simulink subsystem "Torque_Actuated_Configuration_Space_Controller"  (R2021a)
settings: Solver=VariableStepAuto  StartTime=0.0  StopTime=10.0  RelTol=1e-3
undefined symbols (not defined in the file or in its folder): X, Y, Z
libraries: OpenManipulatorLib x5, sm_lib x4, nesl_utility x1
settings Model: Creator=USER  LastModifiedBy=USER

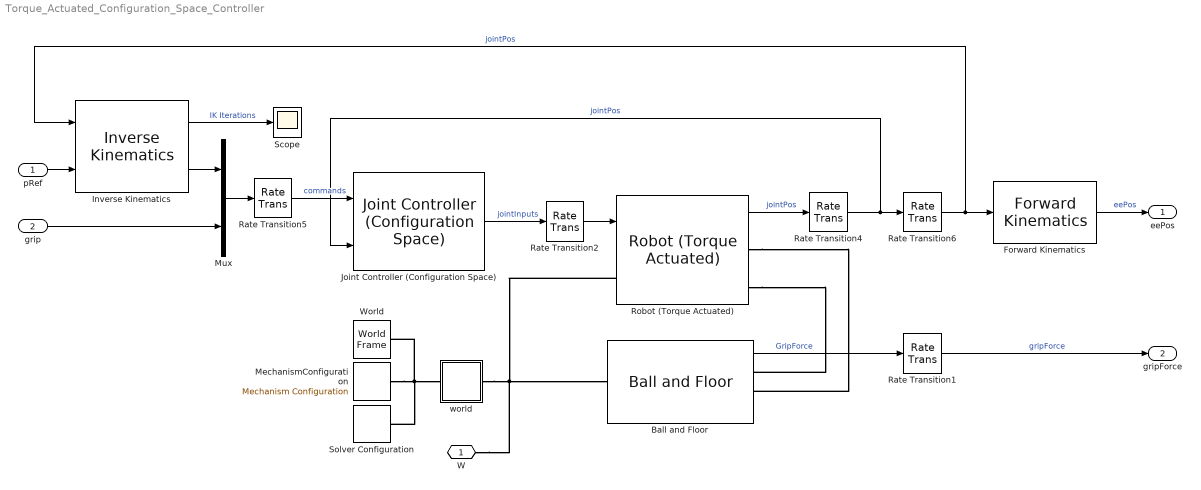
== system Torque_Actuated_Configuration_Space_Controller ==
  "pRef " : Inport
  grip : Inport  Port=2
  Ball and Floor : OpenManipulatorLib/Ball and Floor  PxPositionTargetValue=initPosX  PyPositionTargetValue=initPosY  PxVelocityTargetValue=initVelX  PyVelocityTargetValue=initVelY  PzPositionTargetValue=initPosZ  PzVelocityTargetValue=initVelZ
  Forward Kinematics : OpenManipulatorLib/Forward Kinematics  SystemSampleTime=-1  VariantActivationTime=update diagram  Latency=0  AutoFrameSizeCalculation=off
  Inverse Kinematics : OpenManipulatorLib/Inverse Kinematics  SystemSampleTime=-1  VariantActivationTime=update diagram  Latency=0  AutoFrameSizeCalculation=off
  Joint Controller (Configuration Space) : OpenManipulatorLib/Joint Controller (Configuration Space)  SystemSampleTime=-1  VariantControl=ctrlType==1  VariantActivationTime=update diagram  Latency=0  AutoFrameSizeCalculation=off
  MechanismConfiguration : sm_lib/Utilities/Mechanism Configuration  UniformGravity=Constant  GravityVector=[0 0 -9.80665]  GravityVectorUnits=m/s^2  GravityUnits=m/s^2  LinearizationDelta=0.001  JointModeTransitionNonlinearIterations=2
  Mux : Mux  Inputs=2
  Rate Transition1 : RateTransition
  Rate Transition2 : RateTransition  OutPortSampleTimeOpt=Inherit
  Rate Transition4 : RateTransition
  Rate Transition5 : RateTransition  OutPortSampleTimeOpt=Inherit
  Rate Transition6 : RateTransition
  Robot (Torque Actuated) : OpenManipulatorLib/Robot  (Torque Actuated)  SystemSampleTime=-1  VariantActivationTime=update diagram  Latency=0  AutoFrameSizeCalculation=off
  Scope : Scope
  Solver Configuration : nesl_utility/Solver Configuration  PhysicalDomain=network_engine_domain  SubClassName=solver  LeftPortType=input  RightPortType=generic  Tones=[]  Harmonics=[]  SimulateNoise=off  Profile=off  UseLocalSampling=off  EnableSwitchedLinearOptims=on  FrequencyDomain=off  UseCCode=off  RelTol=0.001  AbsTol=1e-06  MinStep=1e-09  ToWorkspace=off  RevertToSquareIcSolve=off  NumHomotopyIterations=100  PhasorMode=off  PhasorModeNumHarmonics=1  DoDC=off  ResidualTolerance=1e-09  UseLocalSolver=off  LocalSolverChoice=NE_BACKWARD_EULER_ADVANCER  LocalSolverSampleTime=0.001  DoFixedCost=off  MaxNonlinIter=3  MaxModeIter=2  ComputeImpulses=off  ImpulseIterations=2  LinearAlgebra=Sparse  EquationFormulation=NE_TIME_EF  DelaysMemoryBudget=1024  AutomaticFiltering=on  FilteringTimeConstant=0.001  PartitionStorageMethod=AS_NEEDED  PartitionMemoryBudget=1024  PartitionMethod=FAST
  World : sm_lib/Frames and Transforms/World Frame
  world : Subsystem
  W : PMIOPort  Side=Left
  eePos : Outport  VectorParamsAs1DForOutWhenUnconnected=off
  gripForce : Outport  Port=2  VectorParamsAs1DForOutWhenUnconnected=off
  wires:
  Rate Transition5/1 -> Joint Controller (Configuration Space)/1  "commands"
  grip/1 -> Mux/2
  Inverse Kinematics/1 -> Scope/1  "IK Iterations"
  Inverse Kinematics/2 -> Mux/1
  Ball and Floor/1 -> Rate Transition1/1  "GripForce"
  Rate Transition1/1 -> gripForce/1  "gripForce"
  Rate Transition2/1 -> Robot (Torque Actuated)/1
  Joint Controller (Configuration Space)/1 -> Rate Transition2/1  "jointInputs"
  "pRef "/1 -> Inverse Kinematics/2
  Forward Kinematics/1 -> eePos/1  "eePos"
  Robot (Torque Actuated)/1 -> Rate Transition4/1  "jointPos"
  Rate Transition4/1 -> Joint Controller (Configuration Space)/2, Rate Transition6/1  "jointPos"
  Mux/1 -> Rate Transition5/1
  Rate Transition6/1 -> Inverse Kinematics/1, Forward Kinematics/1  "jointPos"
  connections:
  World/RConn1 -- world/LConn1 -- Solver Configuration/RConn1 -- MechanismConfiguration/RConn1
  Robot (Torque Actuated)/LConn1 -- Ball and Floor/LConn1 -- W/RConn1 -- world/RConn1
  Robot (Torque Actuated)/RConn2 -- Ball and Floor/RConn1
  Robot (Torque Actuated)/RConn1 -- Ball and Floor/RConn2

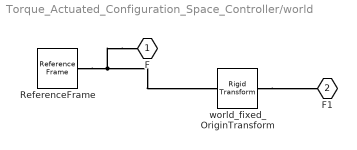
== system Torque_Actuated_Configuration_Space_Controller/world ==
  ReferenceFrame : sm_lib/Frames and Transforms/Reference Frame
  world_fixed_OriginTransform : sm_lib/Frames and Transforms/Rigid Transform  TranslationMethod=Cartesian  TranslationStandardOffset=0  TranslationLengthUnit=m  TranslationStandardAxis=+Z  TranslationCartesianOffset=[0, 0, 0]  TranslationROffset=0  TranslationROffsetUnits=m  TranslationZOffset=0  TranslationZOffsetUnits=m  TranslationThetaOffset=0  TranslationThetaOffsetUnits=deg  RotationMethod=RotationSequence  RotationAngleUnits=deg  RotationStandardAxis=+Z  RotationAngle=0.0  RotationArbitraryAxis=[0 0 1]  FollAlignAxisA=+X  BaseAlignAxisA=+Y  FollAlignAxisB=+Y  BaseAlignAxisB=+Z  RotationSequenceAxes=BaseAxes  RotationSequence=XYZ  RotationSequenceAngles=[0, 0, 0]  RotationSequenceAnglesUnits=rad  RotationMatrix=[1 0 0; 0 1 0; 0 0 1]
  F : PMIOPort  Side=Left
  F1 : PMIOPort  Port=2  Side=Right
  connections:
  world_fixed_OriginTransform/RConn1 -- F1/RConn1
  F/RConn1 -- ReferenceFrame/RConn1 -- world_fixed_OriginTransform/LConn1
